simulink model "Dynamic_without_disturbnce"  (R2018a)
settings: Solver=VariableStepAuto  StartTime=0.0  StopTime=10.0  RelTol=1e-3
values from neighbouring files (symbols this model uses):
  A = double(A)    [Linearization.m]    (also in findK_emtiazi.m = [1 2 0; 0 -1 3; 0 1 -1])
  B = double(B)    [Linearization.m]
  C = [1 0 0 0 ; 0 1 0 0 ]    [Linearization.m]    (also in findK_emtiazi.m = [0 1 0])
  k = place(A,B,pc)    [Linearization.m]
settings Model: Creator=YaCn  LastModifiedBy=YaCn

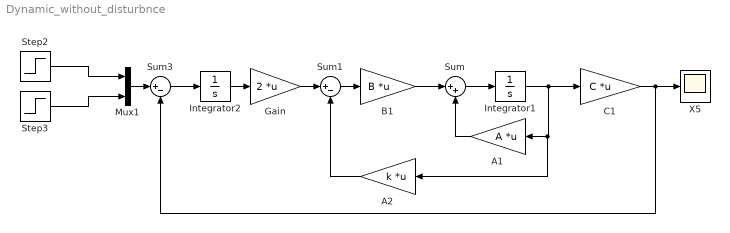
== system Dynamic_without_disturbnce ==
  A1 : Gain  Gain=A  Multiplication=Matrix(K*u) (u vector)
  A2 : Gain  Gain=k  Multiplication=Matrix(K*u) (u vector)
  B1 : Gain  Gain=B  Multiplication=Matrix(K*u) (u vector)
  C1 : Gain  Gain=C  Multiplication=Matrix(K*u) (u vector)
  Gain : Gain  Gain=2  Multiplication=Matrix(K*u)
  Integrator1 : Integrator  InitialCondition=.8
  Integrator2 : Integrator  InitialCondition=0.5
  Mux1 : Mux  Inputs=2
  Step2 : Step  Time=0  SampleTime=0.0001
  Step3 : Step  Time=0  After=1.2  SampleTime=0.001
  Sum : Sum  Inputs=|++
  Sum1 : Sum  Inputs=|+-
  Sum3 : Sum  Inputs=|+-
  X5 : Scope
  wires:
  Sum3/1 -> Integrator2/1
  A2/1 -> Sum1/2
  Gain/1 -> Sum1/1
  Mux1/1 -> Sum3/1
  Integrator2/1 -> Gain/1
  C1/1 -> X5/1, Sum3/2
  Sum1/1 -> B1/1
  Integrator1/1 -> A2/1, A1/1, C1/1
  A1/1 -> Sum/2
  Step2/1 -> Mux1/1
  Step3/1 -> Mux1/2
  Sum/1 -> Integrator1/1
  B1/1 -> Sum/1
